simulink model "UDE_nonlinear"  (R2020a)
settings: Solver=FixedStepAuto  StartTime=0.0  StopTime=tstop  FixedStep=tstep  RelTol=1e-3
values from neighbouring files (symbols this model uses):
  alphaic = [20; 0]    [data.m]
  eic = xic - xmic    [data.m]
  K = place(F_n, G_n, eig(F_m))    [data.m]
  Ts = 0.01    [data.m]
  udic = (-Ts/T)*pinv(G_n)*eic    [data.m]
  xic = [20; 0]    [data.m]
  xmic = [10; 0]    [data.m]
settings Model: Creator=Maithili Shetty  LastModifiedBy=Ram Padmanabhan
settings DataIOCC: ReturnWorkspaceOutputs=off

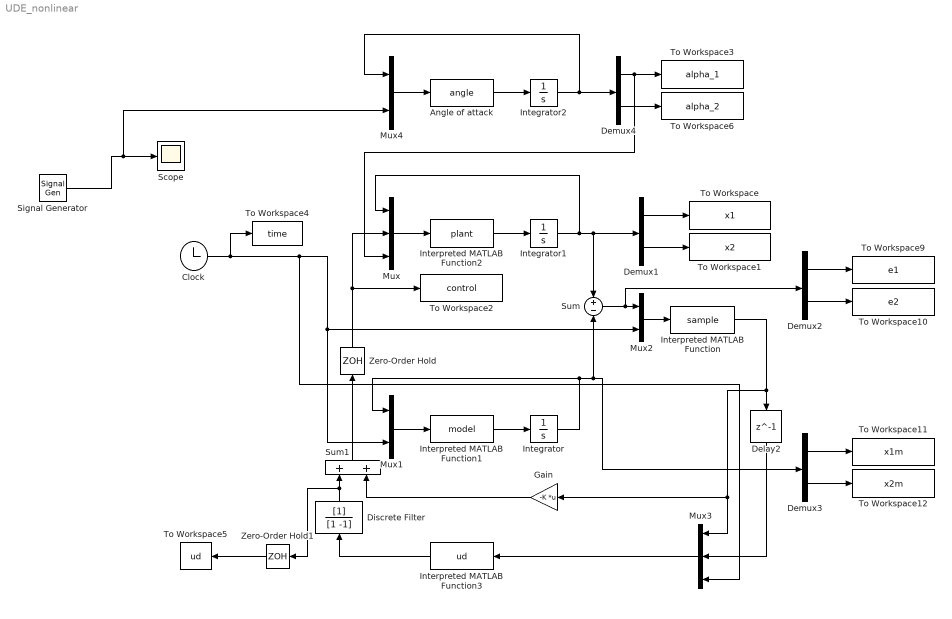
== system UDE_nonlinear ==
  Angle of attack : MATLABFcn  MATLABFcn=angle  OutputDimensions=2
  Clock : Clock
  Delay2 : Delay  DelayLength=1  InitialCondition=eic  SampleTime=Ts
  Demux{1..4} (4 alike) : Demux  Outputs=2
  Discrete Filter : DiscreteFilter  Denominator=[1 -1]  InitialStates=udic  SampleTime=Ts
  Gain : Gain  Gain=-K  Multiplication=Matrix(K*u)
  Integrator : Integrator  InitialCondition=xmic
  Integrator1 : Integrator  InitialCondition=xic
  Integrator2 : Integrator  InitialCondition=alphaic
  Interpreted MATLAB Function : MATLABFcn  MATLABFcn=sample  OutputDimensions=2
  Interpreted MATLAB Function1 : MATLABFcn  MATLABFcn=model  OutputDimensions=2
  Interpreted MATLAB Function2 : MATLABFcn  MATLABFcn=plant  OutputDimensions=2
  Interpreted MATLAB Function3 : MATLABFcn  MATLABFcn=ud  OutputDimensions=1
  Mux : Mux  Inputs=3
  Mux1 : Mux  Inputs=2
  Mux2 : Mux  Inputs=2
  Mux3 : Mux  Inputs=3
  Mux4 : Mux  Inputs=2
  Scope : Scope
  Signal Generator : SignalGenerator  WaveForm=square  Frequency=5  Units=rad/sec
  Sum : Sum  Inputs=+-
  Sum1 : Sum
  To Workspace : ToWorkspace  VariableName=x1  SampleTime=-1
  To Workspace1 : ToWorkspace  VariableName=x2  SampleTime=-1
  To Workspace10 : ToWorkspace  VariableName=e2  SampleTime=-1
  To Workspace11 : ToWorkspace  VariableName=x1m  SampleTime=-1
  To Workspace12 : ToWorkspace  VariableName=x2m  SampleTime=-1
  To Workspace2 : ToWorkspace  VariableName=control  SampleTime=-1
  To Workspace3 : ToWorkspace  VariableName=alpha_1  SampleTime=-1
  To Workspace4 : ToWorkspace  VariableName=time  SampleTime=-1
  To Workspace5 : ToWorkspace  VariableName=ud  SampleTime=-1
  To Workspace6 : ToWorkspace  VariableName=alpha_2  SampleTime=-1
  To Workspace9 : ToWorkspace  VariableName=e1  SampleTime=-1
  Zero-Order Hold : ZeroOrderHold  SampleTime=Ts
  Zero-Order Hold1 : ZeroOrderHold  SampleTime=Ts
  wires:
  Interpreted MATLAB Function3/1 -> Discrete Filter/1
  Interpreted MATLAB Function/1 -> Delay2/1, Mux3/1, Gain/1
  Sum1/1 -> Zero-Order Hold/1
  Discrete Filter/1 -> Zero-Order Hold1/1, Sum1/1
  Mux2/1 -> Interpreted MATLAB Function/1
  Sum/1 -> Demux2/1, Mux2/1
  Mux1/1 -> Interpreted MATLAB Function1/1
  Demux2/1 -> To Workspace9/1
  Demux1/1 -> To Workspace/1
  Integrator/1 -> Demux3/1, Sum/2, Mux1/1
  Mux/1 -> Interpreted MATLAB Function2/1
  Integrator1/1 -> Sum/1, Demux1/1, Mux/1
  Zero-Order Hold1/1 -> To Workspace5/1
  Zero-Order Hold/1 -> To Workspace2/1, Mux/2
  Clock/1 -> Mux3/3, Mux1/2, Mux2/2, To Workspace4/1
  Demux3/2 -> To Workspace12/1
  Interpreted MATLAB Function1/1 -> Integrator/1
  Mux3/1 -> Interpreted MATLAB Function3/1
  Demux3/1 -> To Workspace11/1
  Gain/1 -> Sum1/2
  Demux1/2 -> To Workspace1/1
  Interpreted MATLAB Function2/1 -> Integrator1/1
  Demux2/2 -> To Workspace10/1
  Delay2/1 -> Mux3/2
  Mux4/1 -> Angle of attack/1
  Angle of attack/1 -> Integrator2/1
  Integrator2/1 -> Demux4/1, Mux4/1
  Demux4/1 -> Mux/3, To Workspace3/1
  Demux4/2 -> To Workspace6/1
  Signal Generator/1 -> Mux4/2, Scope/1
